simulink model "TestPosController"  (R2018b)
settings: Solver=VariableStepAuto  StartTime=0.0  StopTime=10.0  RelTol=1e-3
undefined symbols (not defined in the file): INIT_PARAM_VECTOR, mpc_att_sp, mpc_ctrl_state, mpc_manual, mpc_pos_sp_triplet, mpc_vehicle_land_detected, mpc_vehicle_status
libraries: simulink x4
(part 1 of 2)
settings Model: Creator=jban039  LastModifiedBy=jban039
settings SFSimCC: SimUseLocalCustomCode=off
settings RTWCC: RTWUseLocalCustomCode=off
settings CodeAppCC: StateflowObjectComments=on

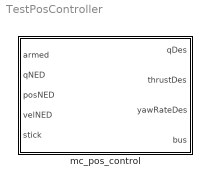
== system TestPosController ==
  mc_pos_control : Subsystem  AncestorBlock=Px4Library/mc_pos_control  mask{THROTTLE_HOVER=0.61703684833922, MPC_SAMPLING_PERIOD=0.02, MPC_THR_MIN=0.12, MPC_THR_HOVER=0.5, MPC_ALTCTL_DZ=0.1, MPC_ALTCTL_DY=0.0, MPC_THR_MAX=0.9, MPC_MANTHR_MIN=0.08, MPC_MANTHR_MAX=0.9, MPC_Z_P=1.0, MPC_Z_VEL_P=0.2, MPC_Z_VEL_I=0.02, MPC_Z_VEL_D=0.0, MPC_Z_VEL_MAX_UP=3.0, MPC_Z_VEL_MAX=1.0, MPC_Z_VEL_MAX_DN=1.0, MPC_Z_FF=0.5, MPC_XY_P=0.95, MPC_XY_VEL_P=0.09, MPC_XY_VEL_I=0.02, MPC_XY_VEL_D=0.01, MPC_XY_CRUISE=5.0, MPC_XY_VEL_MAX=8.0, MPC_XY_FF=0.5, MPC_TILTMAX_AIR=45.0, MPC_TILTMAX_LND=12.0, MPC_LAND_SPEED=0.5, MPC_TKO_SPEED=1.5, MPC_MAN_R_MAX=35.0, MPC_MAN_P_MAX=35.0, MPC_MAN_Y_MAX=200.0, MPC_HOLD_XY_DZ=0.1, MPC_HOLD_MAX_XY=0.8, MPC_HOLD_MAX_Z=0.6, MPC_VELD_LP=5.0, MPC_ACC_HOR_MAX=5.0, MPC_ALT_MODE=0, MC_YAWRATE_MAX=200.0, MC_YAW_P=2.8, VT_OPT_RECOV_EN=0}
      mask init:
      | throttle_hover = THROTTLE_HOVER; % evalin('base', THROTTLE_HOVER);
      | MPC_INIT_SELF = struct( 'mpc_param_find', struct( ...
      | 'MC_YAWRATE_MAX', MC_YAWRATE_MAX, ...
      | 'MC_YAW_P', MC_YAW_P, ...
      | 'MPC_ACC_HOR_MAX', MPC_ACC_HOR_MAX, ...
      | 'MPC_ALTCTL_DY', MPC_ALTCTL_DY, ...
      | 'MPC_ALTCTL_DZ', MPC_ALTCTL_DZ, ...
      | 'MPC_ALT_MODE', MPC_ALT_MODE, ...
      | 'MPC_HOLD_MAX_XY', MPC_HOLD_MAX_XY, ...
      | 'MPC_HOLD_MAX_Z', MPC_HOLD_MAX_Z, ...
      | 'MPC_HOLD_XY_DZ', MPC_HOLD_XY_DZ, ...
      | 'MPC_LAND_SPEED', MPC_LAND_SPEED, ...
      | 'MPC_MAN_P_MAX', MPC_MAN_P_MAX, ...
      | 'MPC_MAN_R_MAX', MPC_MAN_R_MAX, ...
      | 'MPC_MAN_Y_MAX', MPC_MAN_Y_MAX, ...
      | 'MPC_THR_HOVER', MPC_THR_HOVER, ...
      | 'MPC_THR_MAX', MPC_THR_MAX, ...
      | 'MPC_THR_MIN', MPC_THR_MIN, ...
      | 'MPC_TILTMAX_AIR', MPC_TILTMAX_AIR, ...
      | 'MPC_TILTMAX_LND', MPC_TILTMAX_LND, ...
      | 'MPC_TKO_SPEED', MPC_TKO_SPEED, ...
      | 'MPC_XY_CRUISE', MPC_XY_CRUISE, ...
      | 'MPC_XY_FF', MPC_XY_FF, ...
      | 'MPC_XY_P', MPC_XY_P, ...
      | 'MPC_XY_VEL_D', MPC_XY_VEL_D, ...
      | 'MPC_XY_VEL_I', MPC_XY_VEL_I, ...
      | 'MPC_XY_VEL_MAX', MPC_XY_VEL_MAX, ...
      | 'MPC_XY_VEL_P', MPC_XY_VEL_P, ...
      | 'MPC_Z_FF', MPC_Z_FF, ...
      | 'MPC_Z_P', MPC_Z_P, ...
      | 'MPC_Z_VEL_D', MPC_Z_VEL_D, ...
      | 'MPC_Z_VEL_I', MPC_Z_VEL_I, ...
      | 'MPC_Z_VEL_MAX', MPC_Z_VEL_MAX, ...
      | 'MPC_Z_VEL_MAX_DN', MPC_Z_VEL_MAX_DN, ...
      | 'MPC_Z_VEL_MAX_UP', MPC_Z_VEL_MAX_UP, ...
      | 'MPC_Z_VEL_P', MPC_Z_VEL_P, ...
      | 'VT_OPT_RECOV_EN', VT_OPT_RECOV_EN, ...
      | 'MPC_VELD_LP', MPC_VELD_LP ...
      | ), ...
      | 'mpc_thrust_int', [0; 0; -throttle_hover], ...
      | 'mpc_att_sp', struct('thrust', throttle_hover, ...
      | 'q_d', [1; 0; 0; 0;]) ...
      | );

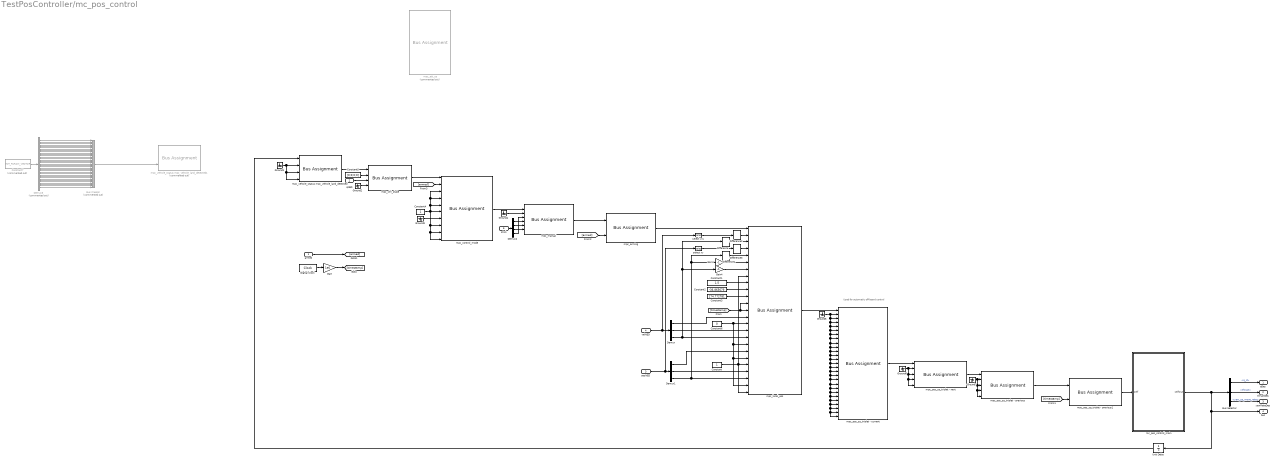
== system TestPosController/mc_pos_control ==
  note: Used for automatic off-board control
  armed : Inport  PortDimensions=1  SampleTime=MPC_SAMPLING_PERIOD
  qNED : Inport  Port=2  PortDimensions=4  SampleTime=MPC_SAMPLING_PERIOD
  posNED : Inport  Port=3  PortDimensions=3  SampleTime=MPC_SAMPLING_PERIOD
  velNED : Inport  Port=4  PortDimensions=3  SampleTime=MPC_SAMPLING_PERIOD
  stick : Inport  Port=5  PortDimensions=4  SampleTime=MPC_SAMPLING_PERIOD
  Bus Creator : BusCreator  Commented=on  Inputs=35  OutDataTypeStr=Bus: mpc_param_find
  Bus Selector : BusSelector  OutputSignals=mpc_att_sp.q_d,mpc_att_sp.thrust,mpc_att_sp.yaw_sp_move_rate
  Constant : Constant  SampleTime=MPC_SAMPLING_PERIOD
  Constant1 : Constant  Value=1.5  SampleTime=MPC_SAMPLING_PERIOD
  Constant2 : Constant  Value=-36.865679  SampleTime=MPC_SAMPLING_PERIOD
  Constant3 : Constant  Value=174.772781  SampleTime=MPC_SAMPLING_PERIOD
  Constant4 : Constant
  Constant5 : Constant  Value=[0;0;0;0]
  Constant6 : Constant  Value=0  SampleTime=MPC_SAMPLING_PERIOD
  Constant7 : Constant  Commented=on  Value=INIT_PARAM_VECTOR
  Demux : Demux  Outputs=3
  Demux1 : Demux  Outputs=3
  Demux2 : Demux
  Demux3 : Demux  Commented=on  Outputs=35
  Difference{,1..3} (4 alike) : simulink/Discrete/Difference  ICPrevInput=0.0  OutMin=[]  OutMax=[]  OutDataType=fixdt(1, 16)  OutScaling=2^-10  DoSatur=off
  Digital Clock : DigitalClock  SampleTime=MPC_SAMPLING_PERIOD
  Gain : Gain  Gain=1e6
  Gain1 : Gain  Gain=-1
  Gain4 : Gain  Gain=-1
  Ground{1..7} (7 alike) : Ground
  Unit Delay : UnitDelay  InitialCondition=MPC_INIT_SELF  SampleTime=MPC_SAMPLING_PERIOD
  mc_pos_control_main : MATLAB Function  TreatAsAtomicUnit=on  SystemSampleTime=MPC_SAMPLING_PERIOD
  mpc_arming : BusAssignment  AssignedSignals=mpc_arming.armed
  mpc_att_sp : BusAssignment  Commented=on  AssignedSignals=mpc_att_sp.disable_mc_yaw_control,mpc_att_sp.landing_gear,mpc_att_sp.pitch_body,mpc_att_sp.q_d,mpc_att_sp.q_d_valid,mpc_att_sp.roll_body,mpc_att_sp.thrust,mpc_att_sp.timestamp,mpc_att_sp.yaw_body,mpc_att_sp.yaw_sp_move_rate
  mpc_control_mode : BusAssignment  AssignedSignals=mpc_control_mode.flag_armed,mpc_control_mode.flag_control_acceleration_enabled,mpc_control_mode.flag_control_altitude_enabled,mpc_control_mode.flag_control_climb_rate_enabled,mpc_control_mode.flag_control_manual_enabled,mpc_control_mode.flag_control_offboard_enabled,mpc_control_mode.flag_control_position_enabled,mpc_control_mode.flag_control_velocity_enabled,mpc_control_mode.flag_control_attitude_enabled
  mpc_ctrl_state : BusAssignment  AssignedSignals=mpc_ctrl_state.delta_q_reset,mpc_ctrl_state.q,mpc_ctrl_state.quat_reset_counter
  mpc_local_pos : BusAssignment  AssignedSignals=mpc_local_pos.delta_vxy,mpc_local_pos.delta_vz,mpc_local_pos.delta_xy,mpc_local_pos.delta_z,mpc_local_pos.dist_bottom,mpc_local_pos.dist_bottom_rate,mpc_local_pos.dist_bottom_valid,mpc_local_pos.ref_alt,mpc_local_pos.ref_lat,mpc_local_pos.ref_lon,mpc_local_pos.ref_timestamp,mpc_local_pos.timestamp,mpc_local_pos.vx,mpc_local_pos.vxy_reset_counter,mpc_local_pos.vy,mpc_local_pos.vz,mpc_local_pos.vz_reset_counter,mpc_local_pos.x,mpc_local_pos.xy_reset_counter,mpc_local_pos.xy_valid,mpc_local_pos.y,mpc_local_pos.z,mpc_local_pos.z_reset_counter,mpc_local_pos.z_valid
  mpc_manual : BusAssignment  AssignedSignals=mpc_manual.gear_switch,mpc_manual.r,mpc_manual.x,mpc_manual.y,mpc_manual.z
  mpc_pos_sp_triplet - current : BusAssignment  AssignedSignals=mpc_pos_sp_triplet.mpc_current.a_x,mpc_pos_sp_triplet.mpc_current.a_y,mpc_pos_sp_triplet.mpc_current.a_z,mpc_pos_sp_triplet.mpc_current.acceleration_valid,mpc_pos_sp_triplet.mpc_current.acceptance_radius,mpc_pos_sp_triplet.mpc_current.alt,mpc_pos_sp_triplet.mpc_current.alt_valid,mpc_pos_sp_triplet.mpc_current.cruising_speed,mpc_pos_sp_triplet.mpc_current.disable_mc_yaw_control,mpc_pos_sp_triplet.mpc_current.lat,mpc_pos_sp_triplet.mpc_current.lon,mpc_pos_sp_triplet.mpc_current.position_valid,mpc_pos_sp_triplet.mpc_current.type,mpc_pos_sp_triplet.mpc_current.valid,mpc_pos_sp_triplet.mpc_current.velocity_frame,mpc_pos_sp_triplet.mpc_current.velocity_valid,mpc_pos_sp_triplet.mpc_current.vx,mpc_pos_sp_triplet.mpc_current.vy,mpc_pos_sp_triplet.mpc_current.vz,mpc_pos_sp_triplet.mpc_current.x,mpc_pos_sp_triplet.mpc_current.y,mpc_pos_sp_triplet.mpc_current.yaw,mpc_pos_sp_triplet.mpc_current.yaw_valid,mpc_pos_sp_triplet.mpc_current.yawspeed,mpc_pos_sp_triplet.mpc_current.yawspeed_valid,mpc_pos_sp_triplet.mpc_current.z
  mpc_pos_sp_triplet - next : BusAssignment  AssignedSignals=mpc_pos_sp_triplet.mpc_next.alt,mpc_pos_sp_triplet.mpc_next.lat,mpc_pos_sp_triplet.mpc_next.lon,mpc_pos_sp_triplet.mpc_next.valid
  mpc_pos_sp_triplet - previous : BusAssignment  AssignedSignals=mpc_pos_sp_triplet.mpc_previous.alt,mpc_pos_sp_triplet.mpc_previous.lat,mpc_pos_sp_triplet.mpc_previous.lon,mpc_pos_sp_triplet.mpc_previous.valid
  mpc_pos_sp_triplet - previous1 : BusAssignment  AssignedSignals=mpc_hrt_absolute_time
  mpc_vehicle_status mpc_vehicle_land_detected : BusAssignment  AssignedSignals=mpc_vehicle_status.is_rotary_wing,mpc_vehicle_status.is_vtol,mpc_vehicle_land_detected.landed
  mpc_vehicle_status mpc_vehicle_land_detected1 : BusAssignment  Commented=on  AssignedSignals=mpc_param_find
  select vxy : Selector  InputPortWidth=3  IndexOptions=Index vector (dialog)  Indices=[1 2]  OutputSizes=1
  select xy : Selector  InputPortWidth=3  IndexOptions=Index vector (dialog)  Indices=[1 2]  OutputSizes=1
  qDes : Outport  PortDimensions=4  SampleTime=MPC_SAMPLING_PERIOD
  thrustDes : Outport  Port=2  PortDimensions=1  SampleTime=MPC_SAMPLING_PERIOD
  yawRateDes : Outport  Port=3  PortDimensions=1  SampleTime=MPC_SAMPLING_PERIOD
  bus : Outport  Port=4  SampleTime=MPC_SAMPLING_PERIOD
  wires:
  Bus Selector/1 -> qDes/1  "<q_d>"
  Bus Selector/2 -> thrustDes/1  "<thrust>"
  Bus Selector/3 -> yawRateDes/1  "<yaw_sp_move_rate>"
  Gain1/1 -> mpc_local_pos/6
  Demux1/3 -> Difference1/1, Gain1/1, mpc_local_pos/23
  Demux3/35 -> Bus Creator/35
  Constant7/1 -> Demux3/1
  Demux3/34 -> Bus Creator/34
  Demux3/33 -> Bus Creator/33
  Demux3/32 -> Bus Creator/32
  Demux3/31 -> Bus Creator/31
  Demux3/30 -> Bus Creator/30
  Demux3/29 -> Bus Creator/29
  Demux3/28 -> Bus Creator/28
  Demux3/27 -> Bus Creator/27
  Demux3/26 -> Bus Creator/26
  Demux3/25 -> Bus Creator/25
  Demux3/24 -> Bus Creator/24
  Demux3/23 -> Bus Creator/23
  Demux3/22 -> Bus Creator/22
  Demux3/21 -> Bus Creator/21
  Demux3/20 -> Bus Creator/20
  Demux3/19 -> Bus Creator/19
  Demux3/18 -> Bus Creator/18
  Demux3/17 -> Bus Creator/17
  Demux3/16 -> Bus Creator/16
  Demux3/15 -> Bus Creator/15
  Demux3/14 -> Bus Creator/14
  Demux3/13 -> Bus Creator/13
  Demux3/12 -> Bus Creator/12
  Demux3/11 -> Bus Creator/11
  Demux3/10 -> Bus Creator/10
  Demux3/9 -> Bus Creator/9
  Demux3/8 -> Bus Creator/8
  Demux3/7 -> Bus Creator/7
  Demux3/6 -> Bus Creator/6
  Demux3/5 -> Bus Creator/5
  Demux3/4 -> Bus Creator/4
  Demux3/3 -> Bus Creator/3
  Demux3/2 -> Bus Creator/2
  Demux3/1 -> Bus Creator/1
  Bus Creator/1 -> mpc_vehicle_status mpc_vehicle_land_detected1/2
  Unit Delay/1 -> mpc_vehicle_status mpc_vehicle_land_detected/1
  Constant5/1 -> mpc_ctrl_state/2
  Demux/3 -> Gain4/1, Difference/1, mpc_local_pos/17
  [armed] -> mpc_control_mode/2
  [armed] -> mpc_arming/2
  armed/1 -> [armed]
  Ground7/1 -> mpc_pos_sp_triplet - previous/2, mpc_pos_sp_triplet - previous/3, mpc_pos_sp_triplet - previous/4, mpc_pos_sp_triplet - previous/5
  Ground6/1 -> mpc_pos_sp_triplet - next/2, mpc_pos_sp_triplet - next/3, mpc_pos_sp_triplet - next/4, mpc_pos_sp_triplet - next/5
  Ground5/1 -> mpc_pos_sp_triplet - current/2, mpc_pos_sp_triplet - current/4, mpc_pos_sp_triplet - current/27, mpc_pos_sp_triplet - current/26, mpc_pos_sp_triplet - current/25, mpc_pos_sp_triplet - current/24, mpc_pos_sp_triplet - current/23, mpc_pos_sp_triplet - current/22, mpc_pos_sp_triplet - current/21, mpc_pos_sp_triplet - current/20, mpc_pos_sp_triplet - current/19, mpc_pos_sp_triplet - current/18, mpc_pos_sp_triplet - current/17, mpc_pos_sp_triplet - current/16, mpc_pos_sp_triplet - current/15, mpc_pos_sp_triplet - current/14, mpc_pos_sp_triplet - current/13, mpc_pos_sp_triplet - current/12, mpc_pos_sp_triplet - current/11, mpc_pos_sp_triplet - current/10, mpc_pos_sp_triplet - current/9, mpc_pos_sp_triplet - current/8, mpc_pos_sp_triplet - current/7, mpc_pos_sp_triplet - current/6, mpc_pos_sp_triplet - current/5, mpc_pos_sp_triplet - current/3
  Demux2/4 -> mpc_manual/3
  Demux2/3 -> mpc_manual/6
  Demux2/2 -> mpc_manual/5
  Demux2/1 -> mpc_manual/4
  stick/1 -> Demux2/1
  Ground4/1 -> mpc_manual/2
  Ground3/1 -> mpc_control_mode/7
  Constant4/1 -> mpc_control_mode/3, mpc_control_mode/4, mpc_control_mode/5, mpc_control_mode/9, mpc_control_mode/10, mpc_control_mode/8, mpc_control_mode/6
  Ground2/1 -> mpc_ctrl_state/4
  Ground1/1 -> mpc_vehicle_status mpc_vehicle_land_detected/2, mpc_vehicle_status mpc_vehicle_land_detected/3, mpc_vehicle_status mpc_vehicle_land_detected/4
  select xy/1 -> Difference3/1
  Difference3/1 -> mpc_local_pos/4
  select vxy/1 -> Difference2/1
  Difference2/1 -> mpc_local_pos/2
  Difference/1 -> mpc_local_pos/3
  Difference1/1 -> mpc_local_pos/5
  Gain4/1 -> mpc_local_pos/7
  Demux1/2 -> mpc_local_pos/22
  Demux1/1 -> mpc_local_pos/19
  posNED/1 -> Demux1/1, select xy/1
  Demux/1 -> mpc_local_pos/14
  Demux/2 -> mpc_local_pos/16
  velNED/1 -> select vxy/1, Demux/1
  Constant2/1 -> mpc_local_pos/10
  Constant3/1 -> mpc_local_pos/11
  Constant1/1 -> mpc_local_pos/9
  [timestamp] -> mpc_pos_sp_triplet - previous1/2
  mpc_pos_sp_triplet - previous1/1 -> mc_pos_control_main/1(self)
  [timestamp] -> mpc_local_pos/13, mpc_local_pos/12
  Gain/1 -> [timestamp]
  Digital Clock/1 -> Gain/1
  Constant/1 -> mpc_local_pos/21, mpc_local_pos/8, mpc_local_pos/25
  Constant6/1 -> mpc_local_pos/15, mpc_local_pos/18, mpc_local_pos/20, mpc_local_pos/24
  mpc_pos_sp_triplet - previous/1 -> mpc_pos_sp_triplet - previous1/1
  mpc_pos_sp_triplet - next/1 -> mpc_pos_sp_triplet - previous/1
  mpc_pos_sp_triplet - current/1 -> mpc_pos_sp_triplet - next/1
  mpc_local_pos/1 -> mpc_pos_sp_triplet - current/1
  mpc_arming/1 -> mpc_local_pos/1
  mpc_manual/1 -> mpc_arming/1
  mpc_ctrl_state/1 -> mpc_control_mode/1
  mpc_control_mode/1 -> mpc_manual/1
  mpc_vehicle_status mpc_vehicle_land_detected/1 -> mpc_ctrl_state/1
  qNED/1 -> mpc_ctrl_state/3
  mc_pos_control_main/1(selfOut) -> Bus Selector/1, bus/1, Unit Delay/1
